simulink model "gm_sampleModel1533_sub_sub"  (R2023a)
settings: Solver=VariableStepAuto  StartTime=0.0  StopTime=10.0  RelTol=1e-3
libraries: hdlsllib x2, simulink x1
settings Model: Creator=user1  LastModifiedBy=user1
settings OptimizationCC: BlockReduction=off  ConditionallyExecuteInputs=off
settings DebuggingCC: InheritedTsInSrcMsg=none

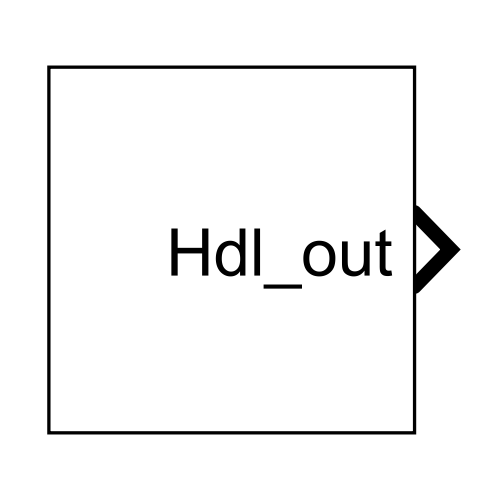
[thumbnail: Simulink's stored preview of the top-level diagram]
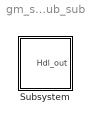
== system gm_sampleModel1533_sub_sub ==
  Subsystem : Subsystem

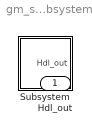
== system gm_sampleModel1533_sub_sub/Subsystem ==
  Subsystem : Subsystem
  Hdl_out : Outport  OutDataTypeStr=uint8

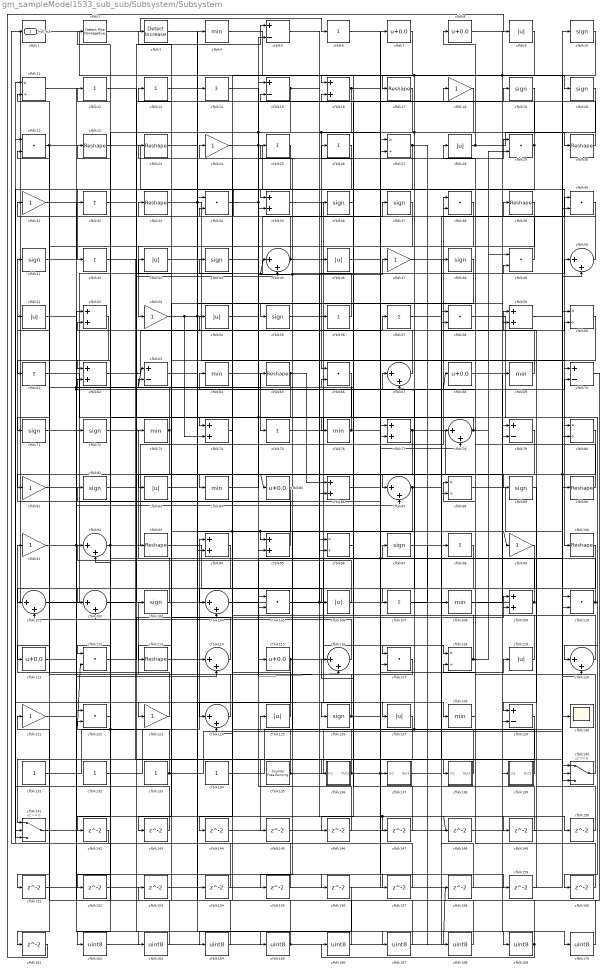
== system gm_sampleModel1533_sub_sub/Subsystem/Subsystem ==
  cfblk1 : ArithShift  BitShiftNumber=8
  cfblk{10,19..20,36..37,41,44,48,55,71..72,82,89,97,103,126} (16 alike) : Signum
  cfblk{17,22..23,30,33,39,65,90,93,100,113} (11 alike) : Reshape
  cfblk{45,50,67,78,87,92,101..102,104,114,116,120,124} (13 alike) : Sum  Inputs=|++  OutDataTypeStr=uint8
  cfblk{21,29,34,38,40,49,58,66,105,110,112,117,122} (13 alike) : DotProduct  OutDataTypeStr=uint8
  cfblk{9,28,43,46,51,54,83,106,119,125,127} (11 alike) : Abs  OutDataTypeStr=uint8  SaturateOnIntegerOverflow=off
  cfblk{6,12..14,25..26,32,42,56..57,61,75,98,107} (14 alike) : Sum  Inputs=+  OutDataTypeStr=uint8
  cfblk{4,64,69,73,76,84,108,128} (8 alike) : MinMax  OutDataTypeStr=uint8
  cfblk{16,35,52,59,62,74,77,86,94..95,109} (11 alike) : Sum  OutDataTypeStr=uint8
  cfblk{11,27,60,80,88,96,118} (7 alike) : Product  Inputs=*/  OutDataTypeStr=uint8  RndMeth=Zero  SaturateOnIntegerOverflow=on
  cfblk{7..8,68,85,111,115} (6 alike) : Bias  Bias=0.0  SaturateOnIntegerOverflow=off
  cfblk{18,24,31,47,53,81,91,99,121,123} (10 alike) : Gain  OutDataTypeStr=uint8
  cfblk{5,15,63,70,79,129} (6 alike) : Sum  Inputs=+-  OutDataTypeStr=uint8
  cfblk130 : Scope
  cfblk{131..134} (4 alike) : Constant  OutDataTypeStr=uint8  SampleTime=-1
  cfblk135 : hdlsllib/Sources/Counter Free-Running  NumBits=16  tsamp=-1
  cfblk136 : Subsystem
      settings: LibrarySourceBlock=|
      | hdlsllib/Ports &
      | Subsystems/Subsystem
  cfblk137 : Subsystem
      settings: LibrarySourceBlock=|
      | hdlsllib/Ports &
      | Subsystems/Subsystem
  cfblk138 : Subsystem
      settings: LibrarySourceBlock=|
      | hdlsllib/Ports &
      | Subsystems/Subsystem
  cfblk139 : Subsystem
      settings: LibrarySourceBlock=|
      | hdlsllib/Ports &
      | Subsystems/Subsystem
  cfblk140 : Switch  OutDataTypeStr=uint8  SaturateOnIntegerOverflow=off  InputSameDT=off
  cfblk141 : Switch  OutDataTypeStr=uint8  SaturateOnIntegerOverflow=off  InputSameDT=off
  cfblk{142..161} (20 alike) : Delay  SampleTime=1
  cfblk{162..170} (9 alike) : DataTypeConversion  OutDataTypeStr=uint8  SaturateOnIntegerOverflow=off  RndMeth=Floor
  cfblk2 : hdlsllib/Logic and Bit Operations/Detect Rise Nonnegative  vinit=0  OutDataTypeStr=uint8
  cfblk3 : simulink/Logic and Bit Operations/Detect Increase  vinit=0.0  OutDataTypeStr=uint8
      settings: LibrarySourceBlock=|
      | hdlsllib/Logic and Bit
      | Operations/Detect
      | Increase
  Hdl_out : Outport  OutDataTypeStr=uint8
  wires:
  cfblk118/1 -> cfblk49/1, cfblk33/1
  cfblk55/1 -> cfblk117/1
  cfblk26/1 -> cfblk35/1
  cfblk1/1 -> cfblk16/1
  cfblk90/1 -> cfblk64/1
  cfblk117/1 -> cfblk103/1
  cfblk45/1 -> cfblk31/1, cfblk128/1
  cfblk140/1 -> cfblk88/1
  cfblk42/1 -> cfblk138/1(In1)
  cfblk40/1 -> cfblk42/1
  cfblk107/1 -> cfblk98/1
  cfblk73/1 -> cfblk142/1, cfblk11/2
  cfblk28/1 -> cfblk8/1, cfblk30/1
  cfblk131/1 -> cfblk14/1
  cfblk91/1 -> cfblk157/1, cfblk37/1
  cfblk80/1 -> cfblk110/2, cfblk85/1
  cfblk18/1 -> cfblk62/1, cfblk66/1
  cfblk84/1 -> cfblk47/1
  cfblk58/1 -> cfblk120/1
  cfblk63/1 -> cfblk95/1, cfblk99/1
  cfblk9/1 -> cfblk74/1, cfblk107/1
  cfblk128/1 -> cfblk28/1
  cfblk2/1 -> cfblk6/1
  cfblk3/1 -> cfblk169/1
  cfblk62/1 -> cfblk86/2, cfblk57/1
  cfblk110/1 -> cfblk160/1, cfblk22/1
  cfblk22/1 -> cfblk100/1
  cfblk33/1 -> cfblk140/3, cfblk55/1
  cfblk46/1 -> cfblk27/1
  cfblk95/1 -> cfblk41/1
  cfblk24/1 -> cfblk106/1, cfblk96/1
  cfblk27/1 -> cfblk168/1, cfblk146/1
  cfblk43/1 -> cfblk96/2
  cfblk53/1 -> cfblk74/2, cfblk89/1, cfblk4/1
  cfblk104/1 -> cfblk97/1
  cfblk94/1 -> cfblk113/1
  cfblk114/1 -> cfblk13/1
  cfblk39/1 -> cfblk53/1
  cfblk132/1 -> cfblk94/1
  cfblk5/1 -> cfblk148/1, cfblk147/1
  cfblk77/1 -> cfblk102/2, cfblk139/1(In1)
  cfblk120/1 -> cfblk59/1
  cfblk13/1 -> cfblk56/1
  cfblk19/1 -> cfblk35/2
  cfblk103/1 -> cfblk73/1
  cfblk123/1 -> cfblk91/1
  cfblk75/1 -> cfblk80/1
  cfblk124/1 -> cfblk21/2
  cfblk92/1 -> cfblk152/1, cfblk38/1
  cfblk138/1(Out1) -> cfblk125/1
  cfblk93/1 -> cfblk105/2
  cfblk105/1 -> cfblk49/2, cfblk10/1
  cfblk8/1 -> cfblk20/1
  cfblk115/1 -> cfblk141/3, cfblk77/2, cfblk79/1
  cfblk134/1 -> cfblk108/1
  cfblk41/1 -> cfblk32/1
  cfblk126/1 -> cfblk70/2, cfblk43/1
  cfblk52/1 -> cfblk61/1
  cfblk64/1 -> cfblk75/1
  cfblk7/1 -> cfblk17/1
  cfblk60/1 -> cfblk83/1
  cfblk102/1 -> cfblk19/1
  cfblk136/1(Out1) -> cfblk25/1, cfblk45/1, cfblk159/1, cfblk119/1
  cfblk109/1 -> Hdl_out/1, cfblk2/1
  cfblk15/1 -> cfblk92/2, cfblk27/2
  cfblk97/1 -> cfblk48/1
  cfblk119/1 -> cfblk66/2
  cfblk108/1 -> cfblk69/1
  cfblk59/1 -> cfblk90/1
  cfblk37/1 -> cfblk101/1
  cfblk54/1 -> cfblk15/1
  cfblk50/1 -> cfblk39/1
  cfblk16/1 -> cfblk78/2, cfblk95/2, cfblk112/1
  cfblk78/1 -> cfblk29/2, cfblk76/1
  cfblk111/1 -> cfblk63/1, cfblk52/1
  cfblk74/1 -> cfblk24/1
  cfblk67/1 -> cfblk54/1
  cfblk137/1(Out1) -> cfblk40/1
  cfblk81/1 -> cfblk68/1, cfblk65/1
  cfblk4/1 -> cfblk140/1
  cfblk85/1 -> cfblk144/1, cfblk143/1
  cfblk35/1 -> cfblk79/2
  cfblk30/1 -> cfblk15/2
  cfblk36/1 -> cfblk126/1
  cfblk113/1 -> cfblk114/1
  cfblk29/1 -> cfblk141/2, cfblk18/1
  cfblk88/1 -> cfblk130/1
  cfblk127/1 -> cfblk141/1
  cfblk125/1 -> cfblk93/1
  cfblk69/1 -> cfblk44/1
  cfblk21/1 -> cfblk156/1, cfblk71/1
  cfblk47/1 -> cfblk88/2
  cfblk133/1 -> cfblk50/2, cfblk62/2, cfblk112/2
  cfblk89/1 -> cfblk129/1
  cfblk141/1 -> cfblk72/1
  cfblk25/1 -> cfblk81/1
  cfblk76/1 -> cfblk51/1, cfblk7/1
  cfblk20/1 -> cfblk124/2, cfblk87/1
  cfblk14/1 -> cfblk70/1
  cfblk23/1 -> cfblk127/1
  cfblk65/1 -> cfblk86/1, cfblk104/1
  cfblk82/1 -> cfblk165/1
  cfblk56/1 -> cfblk23/1
  cfblk72/1 -> cfblk149/1, cfblk5/1
  cfblk86/1 -> cfblk50/1
  cfblk112/1 -> cfblk109/1
  cfblk44/1 -> cfblk29/1
  cfblk12/1 -> cfblk45/2
  cfblk31/1 -> cfblk114/2
  cfblk135/1 -> cfblk52/2, cfblk60/1
  cfblk6/1 -> cfblk118/1
  cfblk139/1(Out1) -> cfblk36/1, cfblk67/1
  cfblk49/1 -> cfblk38/2
  cfblk38/1 -> cfblk84/1
  cfblk17/1 -> cfblk94/2
  cfblk10/1 -> cfblk129/2, cfblk67/2, cfblk46/1
  cfblk100/1 -> cfblk111/1
  cfblk34/1 -> cfblk116/2, cfblk5/2
  cfblk101/1 -> cfblk78/1
  cfblk116/1 -> cfblk101/2
  cfblk71/1 -> cfblk87/2
  cfblk32/1 -> cfblk136/1(In1)
  cfblk106/1 -> cfblk92/1
  cfblk96/1 -> cfblk26/1
  cfblk61/1 -> cfblk115/1, cfblk137/1(In1)
  cfblk99/1 -> cfblk124/1
  cfblk87/1 -> cfblk155/1, cfblk60/2
  cfblk57/1 -> cfblk140/2
  cfblk48/1 -> cfblk123/1
  cfblk66/1 -> cfblk102/1
  cfblk142/1 -> cfblk1/1
  cfblk143/1 -> cfblk11/1
  cfblk144/1 -> cfblk120/2
  cfblk129/1 -> cfblk145/1
  cfblk145/1 -> cfblk80/2
  cfblk146/1 -> cfblk105/1
  cfblk147/1 -> cfblk16/2
  cfblk148/1 -> cfblk40/2
  cfblk149/1 -> cfblk116/1
  cfblk51/1 -> cfblk150/1
  cfblk150/1 -> cfblk59/2
  cfblk79/1 -> cfblk151/1
  cfblk151/1 -> cfblk117/2
  cfblk152/1 -> cfblk110/1
  cfblk70/1 -> cfblk153/1
  cfblk153/1 -> cfblk77/1
  cfblk83/1 -> cfblk154/1
  cfblk154/1 -> cfblk21/1
  cfblk155/1 -> cfblk63/2
  cfblk157/1 -> cfblk104/2
  cfblk158/1 -> cfblk58/1
  cfblk159/1 -> cfblk109/2
  cfblk160/1 -> cfblk118/2
  cfblk98/1 -> cfblk161/1
  cfblk161/1 -> cfblk9/1
  cfblk122/1 -> cfblk162/1
  cfblk162/1 -> cfblk58/2
  cfblk11/1 -> cfblk163/1
  cfblk163/1 -> cfblk122/1
  cfblk156/1 -> cfblk164/1
  cfblk164/1 -> cfblk122/2
  cfblk165/1 -> cfblk12/1, cfblk158/1
  cfblk166/1 -> cfblk82/1
  cfblk121/1 -> cfblk167/1
  cfblk167/1 -> cfblk34/1
  cfblk168/1 -> cfblk121/1
  cfblk169/1 -> cfblk34/2, cfblk166/1
  cfblk68/1 -> cfblk170/1
  cfblk170/1 -> cfblk3/1

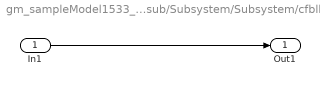
== system gm_sampleModel1533_sub_sub/Subsystem/Subsystem/cfblk136 ==
  In1 : Inport
  Out1 : Outport
  wires:
  In1/1 -> Out1/1

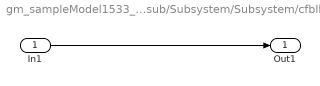
== system gm_sampleModel1533_sub_sub/Subsystem/Subsystem/cfblk137 ==
  In1 : Inport
  Out1 : Outport
  wires:
  In1/1 -> Out1/1

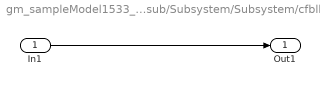
== system gm_sampleModel1533_sub_sub/Subsystem/Subsystem/cfblk138 ==
  In1 : Inport
  Out1 : Outport
  wires:
  In1/1 -> Out1/1

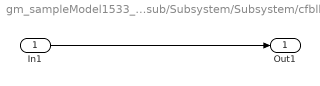
== system gm_sampleModel1533_sub_sub/Subsystem/Subsystem/cfblk139 ==
  In1 : Inport
  Out1 : Outport
  wires:
  In1/1 -> Out1/1
